simulink model "ElectricCircuitWithInitialConditions"  (R2019b)
settings: Solver=VariableStepAuto  StartTime=0.0  StopTime=10.0  RelTol=1e-3
settings Model: Creator=Lenovo  LastModifiedBy=Lenovo

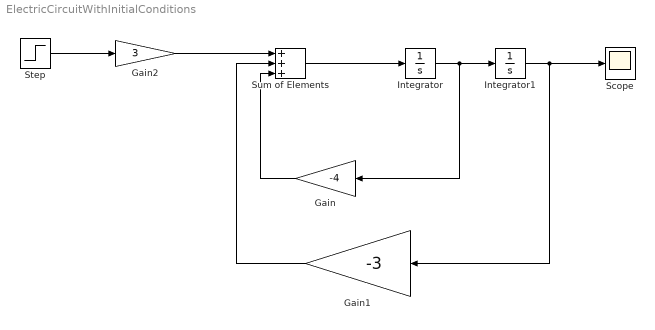
== system ElectricCircuitWithInitialConditions ==
  Gain : Gain  Gain=-4
  Gain1 : Gain  Gain=-3
  Gain2 : Gain  Gain=3
  Integrator : Integrator
  Integrator1 : Integrator  InitialCondition=0.5
  Scope : Scope
  Step : Step  SampleTime=0
  Sum of Elements : Sum  Inputs=+++
  wires:
  Sum of Elements/1 -> Integrator/1
  Gain/1 -> Sum of Elements/3
  Integrator/1 -> Gain/1, Integrator1/1
  Gain1/1 -> Sum of Elements/2
  Integrator1/1 -> Scope/1, Gain1/1
  Gain2/1 -> Sum of Elements/1
  Step/1 -> Gain2/1
